simulink model "network_armax"  (R2024a)
settings: Solver=FixedStepDiscrete  StartTime=0.0  StopTime=499  FixedStep=1  RelTol=1e-3
values from neighbouring files (symbols this model uses):
  theta = [1 0.25 0.3 0.15 0.3 -0.01 -0.8 0.15 0.8 -0.3 -0.8 0.2 ... (42 elements, 1x42)]    [Copy_of_true_system.mat]    (also in a_generate_stable_system.m = [A1(2:3)' B1' C1(2:3)' A2(2:3)' B2' C2(2:3)' A3(2:3)' B3' C3)
settings Model: Creator=jogal  LastModifiedBy=jogal
settings OptimizationCC: ReuseModelBlockBuffer=off
settings RTWCC: GPUComputeCapability=3.5

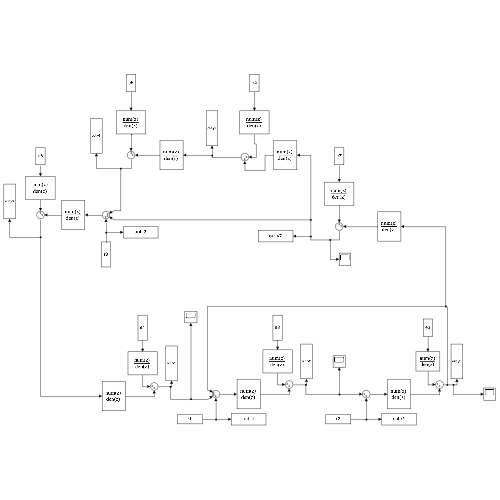
[thumbnail: Simulink's stored preview of the top-level diagram]
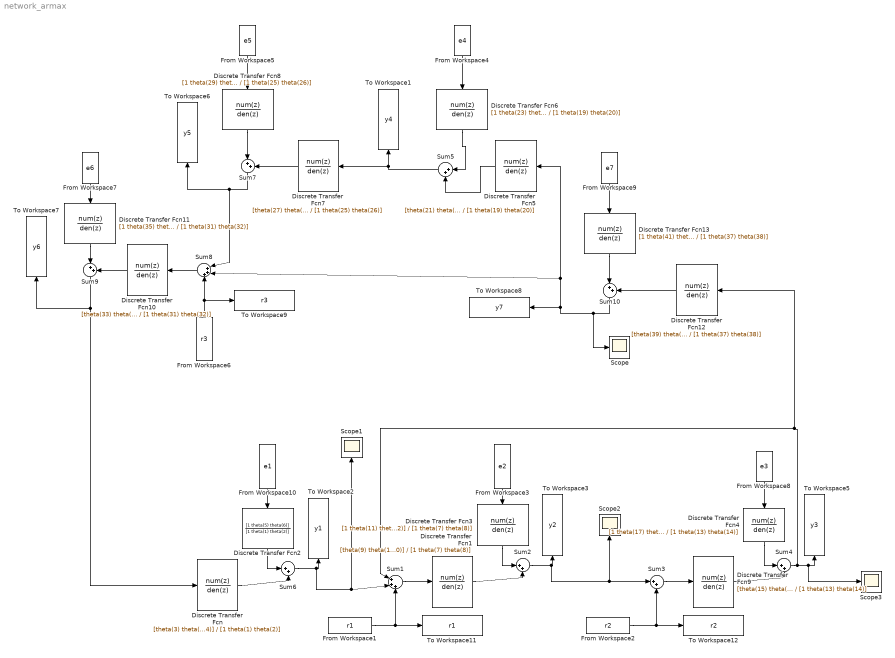
== system network_armax ==
  Discrete Transfer Fcn : DiscreteTransferFcn  Numerator=[theta(3) theta(4)]  Denominator=[1 theta(1) theta(2)]
  Discrete Transfer Fcn1 : DiscreteTransferFcn  Numerator=[theta(9) theta(10)]  Denominator=[1 theta(7) theta(8)]
  Discrete Transfer Fcn10 : DiscreteTransferFcn  Numerator=[theta(33) theta(34)]  Denominator=[1 theta(31) theta(32)]
  Discrete Transfer Fcn11 : DiscreteTransferFcn  Numerator=[1 theta(35) theta(36)]  Denominator=[1 theta(31) theta(32)]
  Discrete Transfer Fcn12 : DiscreteTransferFcn  Numerator=[theta(39) theta(40)]  Denominator=[1 theta(37) theta(38)]
  Discrete Transfer Fcn13 : DiscreteTransferFcn  Numerator=[1 theta(41) theta(42)]  Denominator=[1 theta(37) theta(38)]
  Discrete Transfer Fcn2 : DiscreteTransferFcn  Numerator=[1 theta(5) theta(6)]  Denominator=[1 theta(1) theta(2)]
  Discrete Transfer Fcn3 : DiscreteTransferFcn  Numerator=[1 theta(11) theta(12)]  Denominator=[1 theta(7) theta(8)]
  Discrete Transfer Fcn4 : DiscreteTransferFcn  Numerator=[1 theta(17) theta(18)]  Denominator=[1 theta(13) theta(14)]
  Discrete Transfer Fcn5 : DiscreteTransferFcn  Numerator=[theta(21) theta(22)]  Denominator=[1 theta(19) theta(20)]
  Discrete Transfer Fcn6 : DiscreteTransferFcn  Numerator=[1 theta(23) theta(24)]  Denominator=[1 theta(19) theta(20)]
  Discrete Transfer Fcn7 : DiscreteTransferFcn  Numerator=[theta(27) theta(28)]  Denominator=[1 theta(25) theta(26)]
  Discrete Transfer Fcn8 : DiscreteTransferFcn  Numerator=[1 theta(29) theta(30)]  Denominator=[1 theta(25) theta(26)]
  Discrete Transfer Fcn9 : DiscreteTransferFcn  Numerator=[theta(15) theta(16)]  Denominator=[1 theta(13) theta(14)]
  From Workspace1 : FromWorkspace  VariableName=r1  SampleTime=1  Interpolate=off  OutputAfterFinalValue=Holding final value
  From Workspace10 : FromWorkspace  VariableName=e1  SampleTime=1  Interpolate=off  OutputAfterFinalValue=Holding final value
  From Workspace2 : FromWorkspace  VariableName=r2  SampleTime=1  Interpolate=off  OutputAfterFinalValue=Holding final value
  From Workspace3 : FromWorkspace  VariableName=e2  SampleTime=1  Interpolate=off  OutputAfterFinalValue=Holding final value
  From Workspace4 : FromWorkspace  VariableName=e4  SampleTime=1  Interpolate=off  OutputAfterFinalValue=Holding final value
  From Workspace5 : FromWorkspace  VariableName=e5  SampleTime=1  Interpolate=off  OutputAfterFinalValue=Holding final value
  From Workspace6 : FromWorkspace  VariableName=r3  SampleTime=1  Interpolate=off  OutputAfterFinalValue=Holding final value
  From Workspace7 : FromWorkspace  VariableName=e6  SampleTime=1  Interpolate=off  OutputAfterFinalValue=Holding final value
  From Workspace8 : FromWorkspace  VariableName=e3  SampleTime=1  Interpolate=off  OutputAfterFinalValue=Holding final value
  From Workspace9 : FromWorkspace  VariableName=e7  SampleTime=1  Interpolate=off  OutputAfterFinalValue=Holding final value
  Scope{,1..3} (4 alike) : Scope
  Sum1 : Sum  Inputs=|+++
  Sum{2..7,9..10} (8 alike) : Sum  Inputs=|++
  Sum8 : Sum  Inputs=|+++
  To Workspace1 : ToWorkspace  VariableName=y4  SampleTime=-1
  To Workspace11 : ToWorkspace  VariableName=r1  SampleTime=-1
  To Workspace12 : ToWorkspace  VariableName=r2  SampleTime=-1
  To Workspace2 : ToWorkspace  VariableName=y1  SampleTime=-1
  To Workspace3 : ToWorkspace  VariableName=y2  SampleTime=-1
  To Workspace5 : ToWorkspace  VariableName=y3  SampleTime=-1
  To Workspace6 : ToWorkspace  VariableName=y5  SampleTime=-1
  To Workspace7 : ToWorkspace  VariableName=y6  SampleTime=-1
  To Workspace8 : ToWorkspace  VariableName=y7  SampleTime=-1
  To Workspace9 : ToWorkspace  VariableName=r3  SampleTime=-1
  wires:
  Sum9/1 -> Discrete Transfer Fcn/1, To Workspace7/1
  Sum6/1 -> Sum1/2, Scope1/1, To Workspace2/1
  From Workspace10/1 -> Discrete Transfer Fcn2/1
  From Workspace8/1 -> Discrete Transfer Fcn4/1
  Discrete Transfer Fcn/1 -> Sum6/2
  Discrete Transfer Fcn2/1 -> Sum6/1
  From Workspace3/1 -> Discrete Transfer Fcn3/1
  From Workspace1/1 -> Sum1/3, To Workspace11/1
  Sum1/1 -> Discrete Transfer Fcn1/1
  Discrete Transfer Fcn1/1 -> Sum2/2
  Discrete Transfer Fcn3/1 -> Sum2/1
  Discrete Transfer Fcn9/1 -> Sum4/2
  From Workspace2/1 -> To Workspace12/1, Sum3/2
  Sum3/1 -> Discrete Transfer Fcn9/1
  Sum4/1 -> Discrete Transfer Fcn12/1, Sum1/1, Scope3/1, To Workspace5/1
  Sum2/1 -> Scope2/1, Sum3/1, To Workspace3/1
  Discrete Transfer Fcn4/1 -> Sum4/1
  From Workspace4/1 -> Discrete Transfer Fcn6/1
  From Workspace5/1 -> Discrete Transfer Fcn8/1
  Discrete Transfer Fcn5/1 -> Sum5/2
  Discrete Transfer Fcn6/1 -> Sum5/1
  Discrete Transfer Fcn7/1 -> Sum7/2
  Discrete Transfer Fcn8/1 -> Sum7/1
  Sum5/1 -> To Workspace1/1, Discrete Transfer Fcn7/1
  Sum7/1 -> Sum8/1, To Workspace6/1
  From Workspace6/1 -> To Workspace9/1, Sum8/3
  Sum8/1 -> Discrete Transfer Fcn10/1
  Discrete Transfer Fcn10/1 -> Sum9/2
  Discrete Transfer Fcn11/1 -> Sum9/1
  From Workspace7/1 -> Discrete Transfer Fcn11/1
  From Workspace9/1 -> Discrete Transfer Fcn13/1
  Discrete Transfer Fcn13/1 -> Sum10/1
  Discrete Transfer Fcn12/1 -> Sum10/2
  Sum10/1 -> Scope/1, Sum8/2, Discrete Transfer Fcn5/1, To Workspace8/1
